simulink subsystem "starTracker"  (R2023b)
settings: Solver=VariableStepAuto  StartTime=0.0  StopTime=10.0  RelTol=1e-3
undefined symbols (not defined in the file or in its folder): starTracker
libraries: sensors_subsystems x4, dyn_lib x1
settings Model: DataDictionary=SimulationDict.sldd  EnableAccessToBaseWorkspace=off  Creator=brent  LastModifiedBy=brent

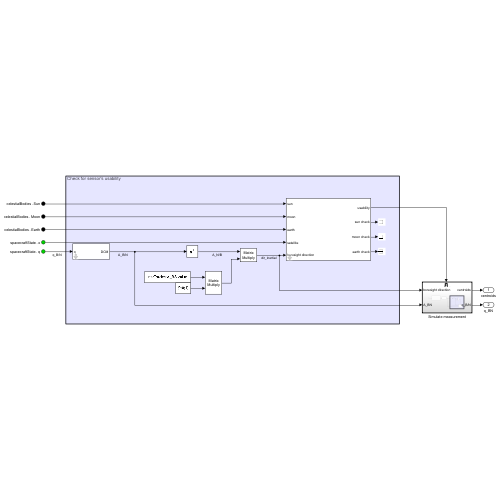
[thumbnail: Simulink's stored preview of the top-level diagram]
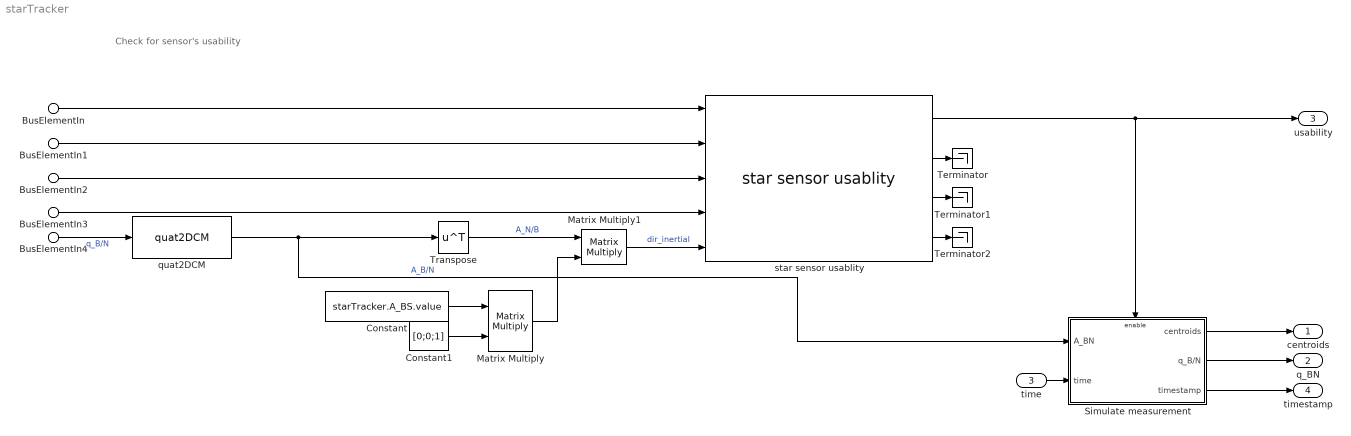
== system starTracker ==
  note: Check for sensor's usability
  BusElementIn : Inport  PortName=celestialBodies  Element=Sun
  BusElementIn2 : Inport  PortName=celestialBodies  Element=Earth
  BusElementIn1 : Inport  PortName=celestialBodies  Element=Moon
  BusElementIn3 : Inport  Port=2  PortName=spacecraftState  Element=x
  BusElementIn4 : Inport  Port=2  PortName=spacecraftState  Element=q
  time : Inport  Port=3
  Constant : Constant  Value=starTracker.A_BS.value
  Constant1 : Constant  Value=[0;0;1]
  Matrix Multiply : Product  Multiplication=Matrix(*)
  Matrix Multiply1 : Product  Multiplication=Matrix(*)
  Simulate measurement : Subsystem  TreatAsAtomicUnit=on
  Terminator : Terminator
  Terminator1 : Terminator
  Terminator2 : Terminator
  Transpose : Math  Operator=transpose
  quat2DCM : dyn_lib/quat2DCM
      settings: SourceProductName=Dynamics library
  star sensor usablity : sensors_subsystems/star sensor usablity  R_M=Environment.Moon.radius.value  R_E=Environment.Earth.radius.value  exclusionAngle=starTracker.exclusionAngle.value  fov=starTracker.fov.value
      settings: SourceProductName=Sensors library
  centroids : Outport
  q_BN : Outport  Port=2
  usability : Outport  Port=3
  timestamp : Outport  Port=4
  wires:
  BusElementIn/1 -> star sensor usablity/1
  BusElementIn1/1 -> star sensor usablity/2
  BusElementIn2/1 -> star sensor usablity/3
  BusElementIn3/1 -> star sensor usablity/4
  star sensor usablity/2 -> Terminator/1
  star sensor usablity/3 -> Terminator1/1
  star sensor usablity/4 -> Terminator2/1
  star sensor usablity/1 -> usability/1, Simulate measurement/Enable
  BusElementIn4/1 -> quat2DCM/1  "q_B/N"
  quat2DCM/1 -> Transpose/1, Simulate measurement/1(A_BN)  "A_B/N"
  Transpose/1 -> Matrix Multiply1/1  "A_N/B"
  Constant/1 -> Matrix Multiply/1
  Constant1/1 -> Matrix Multiply/2
  Matrix Multiply/1 -> Matrix Multiply1/2
  Matrix Multiply1/1 -> star sensor usablity/5  "dir_inertial"
  Simulate measurement/1(centroids) -> centroids/1
  Simulate measurement/2(q_B/N) -> q_BN/1
  time/1 -> Simulate measurement/2(time)
  Simulate measurement/3(timestamp) -> timestamp/1

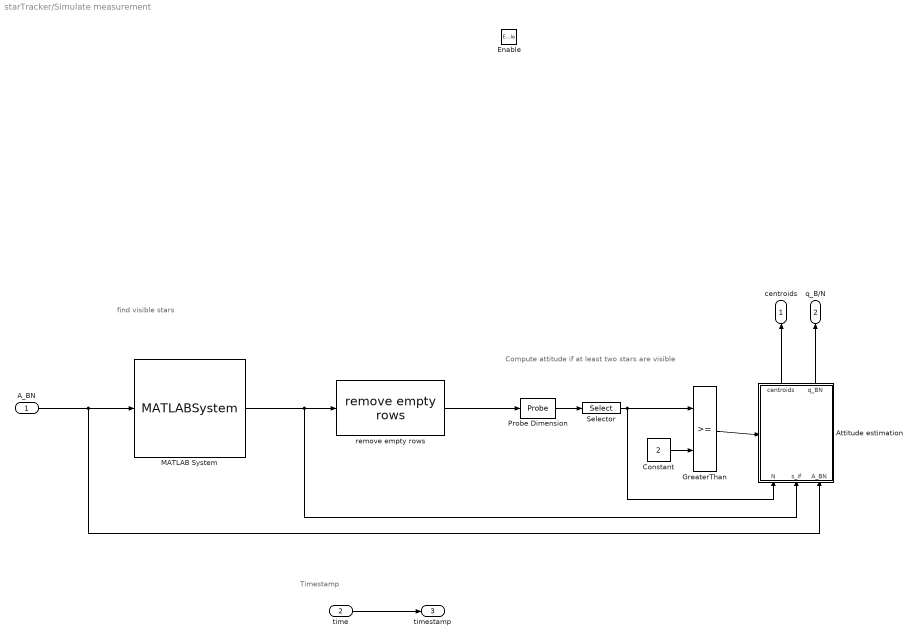
== system starTracker/Simulate measurement ==
  note: Compute attitude if at least two stars are visible
  note: find visible stars
  note: Timestamp
  A_BN : Inport
  time : Inport  Port=2
  Enable : EnablePort  PropagateVarSize=During execution
  Attitude estimation : Subsystem  TreatAsAtomicUnit=on
  Constant : Constant  Value=2
  GreaterThan : RelationalOperator  OutDataTypeStr=boolean  RndMeth=Simplest  InputSameDT=off
  MATLAB System : MATLABSystem  System=visibleStars  starTracker=starTracker  SimulateUsing=Code generation
      mask Type: visibleStars
      mask Display:
      | disp('visibleStars');
      | port_label('input',1,'A_BN');
      | port_label('output',1,'s_if');
  Probe Dimension : Probe  ProbeWidth=off  ProbeSampleTime=off  ProbeComplexSignal=off  ProbeSignalDimensions=on
  Selector : Selector  InputPortWidth=2  IndexOptions=Index vector (dialog)  Indices=1  OutputSizes=1
  remove empty rows : sensors_subsystems/remove empty rows
      settings: SourceProductName=Sensors library
  centroids : Outport
  q_B/N : Outport  Port=2
  timestamp : Outport  Port=3
  wires:
  time/1 -> timestamp/1
  Selector/1 -> Attitude estimation/1(N), GreaterThan/1
  MATLAB System/1 -> remove empty rows/1, Attitude estimation/2(s_if)
  remove empty rows/1 -> Probe Dimension/1
  Probe Dimension/1 -> Selector/1
  Constant/1 -> GreaterThan/2
  GreaterThan/1 -> Attitude estimation/Enable
  A_BN/1 -> MATLAB System/1, Attitude estimation/3(A_BN)
  Attitude estimation/1(centroids) -> centroids/1
  Attitude estimation/2(q_BN) -> q_B/N/1

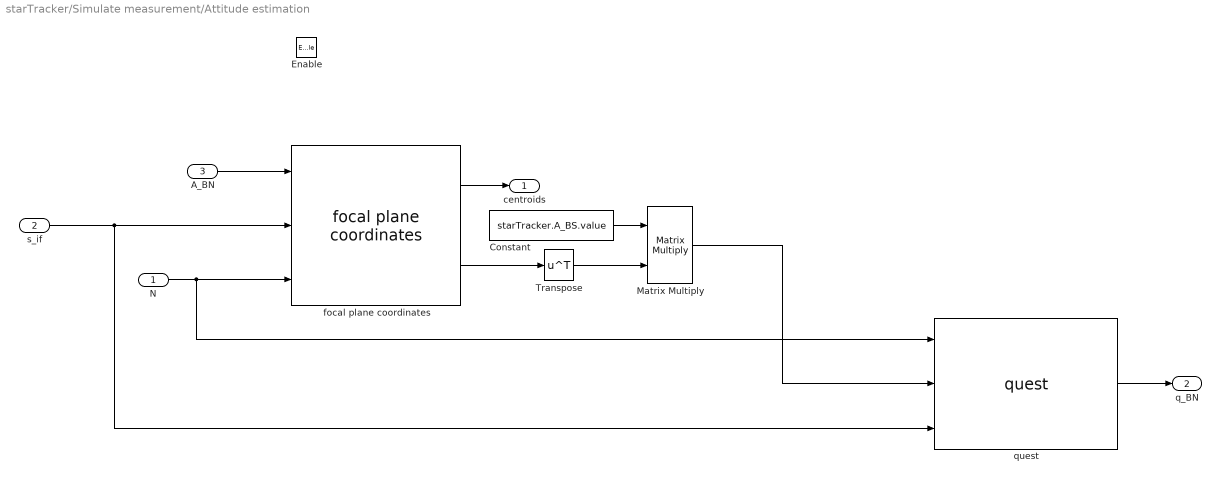
== system starTracker/Simulate measurement/Attitude estimation ==
  N : Inport
  s_if : Inport  Port=2
  A_BN : Inport  Port=3
  Enable : EnablePort
  Constant : Constant  Value=starTracker.A_BS.value
  Matrix Multiply : Product  Multiplication=Matrix(*)
  Transpose : Math  Operator=transpose
  focal plane coordinates : sensors_subsystems/focal plane coordinates  starTracker=starTracker  mag_seed=abs(round(rand(1)*1e4))  angle_seed=abs(round(rand(1)*1e4))
      settings: SourceProductName=Sensors library
  quest : sensors_subsystems/quest
      settings: SourceProductName=Sensors library
  centroids : Outport
  q_BN : Outport  Port=2
  wires:
  quest/1 -> q_BN/1
  Transpose/1 -> Matrix Multiply/2
  s_if/1 -> quest/3, focal plane coordinates/2
  focal plane coordinates/1 -> centroids/1
  A_BN/1 -> focal plane coordinates/1
  Matrix Multiply/1 -> quest/2
  focal plane coordinates/2 -> Transpose/1
  Constant/1 -> Matrix Multiply/1
  N/1 -> focal plane coordinates/3, quest/1
